simulink model "test_1"  (R2016b)
settings: Solver=VariableStepAuto  StartTime=0.0  StopTime=30  FixedStep=1e-4  MaxStep=1e-3  RelTol=1e-6
values from neighbouring files (symbols this model uses):
  K = dlqr(lipm_d.A, lipm_d.B, diag([0 1 1]), 0.0001)    [setup_variables.m]
settings Model: Creator=arturo  LastModifiedBy=arturo

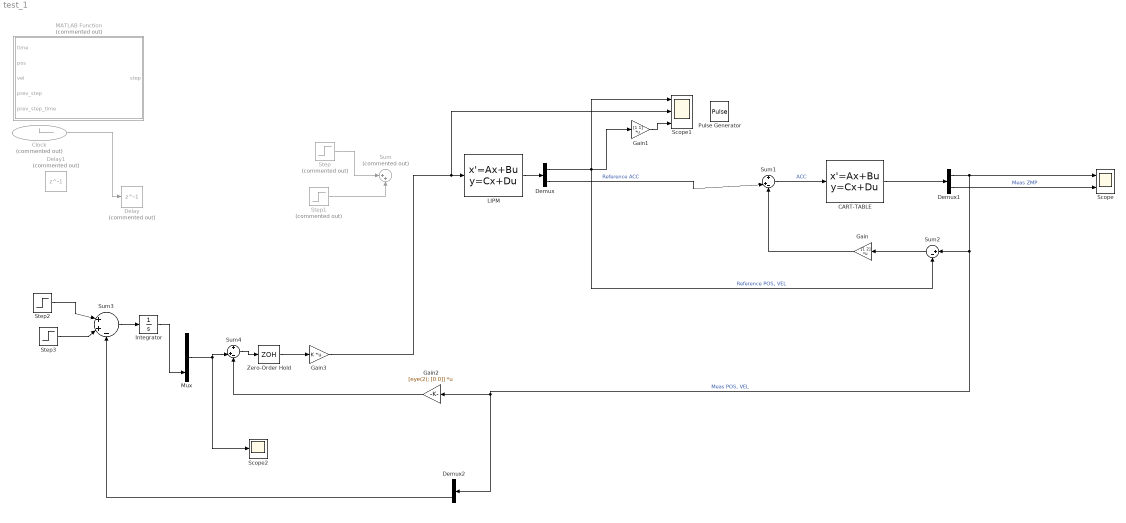
== system test_1 ==
  CART-TABLE : StateSpace  A=[0 1; 0 0]  B=[0; 1]  C=[eye(2); [1 0]]  D=[0; 0; -1]  X0=[0 0]
  Clock : Clock  Commented=on
  Delay : Delay  Commented=on  DelayLength=1  InitialCondition=0
  Delay1 : Delay  Commented=on  DelayLength=1  InitialCondition=0
  Demux : Demux  Outputs=[2 1]
  Demux1 : Demux  Outputs=[2 1]
  Demux2 : Demux  Outputs=[1 1]
  Gain : Gain  Gain=[1 2]  Multiplication=Matrix(K*u)
  Gain1 : Gain  Gain=[1 1]  Multiplication=Matrix(K*u)
  Gain2 : Gain  Gain=[eye(2); [0 0]]  Multiplication=Matrix(K*u)
  Gain3 : Gain  Gain=K  Multiplication=Matrix(K*u)
  Integrator : Integrator
  LIPM : StateSpace  A=[0 1; 1 0]  B=[0; -1]  C=[eye(2); [1 0]]  D=[0; 0; -1]  X0=[0 0]
  MATLAB Function : MATLAB Function  Commented=on  TreatAsAtomicUnit=on
  Mux : Mux  Inputs=3
  Pulse Generator : DiscretePulseGenerator  PulseType=Time based  PulseWidth=5
  Scope : Scope  NumInputPorts=2
  Scope1 : Scope  NumInputPorts=3
  Scope2 : Scope
  Step : Step  Commented=on  After=-exp(-1)  SampleTime=0
  Step1 : Step  Commented=on  Time=2  SampleTime=0
  Step2 : Step  Time=10  SampleTime=0
  Step3 : Step  Time=20  After=-1  SampleTime=0
  Sum : Sum  Commented=on  Inputs=|++
  Sum1 : Sum  Inputs=+|+-
  Sum2 : Sum  Inputs=|+-
  Sum3 : Sum  Inputs=|++-
  Sum4 : Sum  Inputs=+|+-
  Zero-Order Hold : ZeroOrderHold
  wires:
  Step/1 -> Sum/1
  Step1/1 -> Sum/2
  Sum1/1 -> CART-TABLE/1  "ACC"
  Sum2/1 -> Gain/1
  LIPM/1 -> Demux/1
  Demux/1 -> Gain1/1, Sum2/2, Scope1/1  "Reference POS, VEL"
  CART-TABLE/1 -> Demux1/1
  Demux1/1 -> Gain2/1, Demux2/1, Sum2/1, Scope/1  "Meas POS, VEL"
  Demux/2 -> Sum1/2  "Reference ACC"
  Demux1/2 -> Scope/2  "Meas ZMP"
  Clock/1 -> Delay/1
  Gain/1 -> Sum1/3
  Gain1/1 -> Scope1/3
  Gain3/1 -> Scope1/2, LIPM/1
  Zero-Order Hold/1 -> Gain3/1
  Sum4/1 -> Zero-Order Hold/1
  Step2/1 -> Sum3/1
  Step3/1 -> Sum3/2
  Mux/1 -> Scope2/1, Sum4/2
  Demux2/2 -> Sum3/3
  Sum3/1 -> Integrator/1
  Integrator/1 -> Mux/3
  Gain2/1 -> Sum4/3

== matlab function test_1/MATLAB Function ==
  data: time input; step output; pos input; vel input; prev_step input; prev_step_time input
function step = footstep_planning(time, pos, vel, prev_step, prev_step_time)

% pos + vel =  p_0 + s_1*e^(t1) + s_2*e^(t2) + ...

n_steps = 5;
future_ts = 0:(n_steps-1); %ceil(time):(floor(time)+5);
exp_ts = exp(-future_ts);

A = [exp_ts; ones(1, n_steps)];
b = [0 + 0.4; 1];

s = pinv(A)*b;

steps = cumsum(s);


if time == floor(time) && time < 5
    
    step = steps(floor(time)+1);
    
%     future_ts = 0:(n_steps-1); %ceil(time):(floor(time)+5);
%     exp_ts = exp(-future_ts);
%     
%     
%     A = [exp_ts; ones(1, n_steps)];
%     b = [0 + vel; 1];
%     
%     s = pinv(A)*b;
%     
%     step = prev_step + s(1);
    
else
    
    step = prev_step;
    
end
